simulink model "hydraulic_actuator"  (R2019b)
settings: Solver=ode23t  StartTime=0.0  StopTime=10.0  MaxStep=0.001  RelTol=1e-6  EnableMultiTasking=on
libraries: simulink x1
Description:
  | Closed-Loop Electrohydraulic Actuator with Proportional Valve
  | 
  | This example shows an actuator that consists of a proportional 4-way directional valve
  | driving a double-acting hydraulic cylinder. The cylinder drives a load consisting of a mass,
  | viscous and Coulomb friction, constant force, and a spring. The actuator is powered
  | by a variable-displacement, pressure-compensated pump, driven by a constant velocity
  | motor. Pipelines between the valve, cylinder, pump, and the tank are simulated
  | with the Hydraulic Pipeline blocks.
  | 
  | 
  | Copyright 2008-2013 The MathWorks, Inc.
settings Model: DataDictionary=HeliSystemDD.sldd  ExtModeAutoUpdateStatusClock=off  Creator=MathWorks  LastModifiedBy=bpotter
settings DataIOCC: LimitDataPoints=on  SaveFormat=Array  SaveOutput=off  SignalLogging=off  DSMLogging=off  SaveTime=off  ReturnWorkspaceOutputs=off
settings OptimizationCC: DefaultParameterBehavior=Inlined  UseDivisionForNetSlopeComputation=on  ExpressionDepthLimit=2147483647  InitFltsAndDblsToZero=on  LifeSpan=inf
settings DebuggingCC: SaveWithParameterizedLinksMsg=none  SignalResolutionControl=TryResolveAllWithWarning  SolverPrmCheckMsg=warning  MultiTaskDSMMsg=warning  ParameterPrecisionLossMsg=none  AllowSymbolicDim=off  StateNameClashWarn=warning  PregeneratedLibrarySubsystemCodeDiagnostic=none  StrictBusMsg=ErrorOnBusTreatedAsVector  NonBusSignalsTreatedAsBus=error  SFUnexpectedBacktrackingDiag=warning  SFNoUnconditionalDefaultTransitionDiag=warning  SFExecutionAtInitializationDiag=none  ArithmeticOperatorsInVariantConditions=warning
settings HardwareCC: ProdBitPerPointer=32  ProdBitPerSizeT=32  ProdBitPerPtrDiffT=32  ProdLargestAtomicFloat=None  ProdEndianess=Unspecified  ProdWordSize=32  ProdHWDeviceType=32-bit Generic
settings ModelReferenceCC: PropagateSignalLabelsOutOfModel=off
settings SFSimCC: SimUseLocalCustomCode=off  CustomCodeUndefinedFunction=UseInterfaceOnly
settings RTWCC: RTWUseLocalCustomCode=off
settings CodeAppCC: StateflowObjectComments=on
settings GRTTargetCC: TargetFcnLib=ansi_tfl_tmw.mat  TargetLangStandard=C89/C90 (ANSI)  GeneratePreprocessorConditionals=Disable all  CombineOutputUpdateFcns=off  GRTInterface=on
settings ConfigComp: CovMetricSettings=dw  CovHtmlReporting=on  CovSaveCumulativeToWorkspaceVar=on  CovSaveSingleToWorkspaceVar=on  CovExternalEMLEnable=off  CovSFcnEnable=off
settings SimscapeCC: SimscapeNormalizeSystem=off

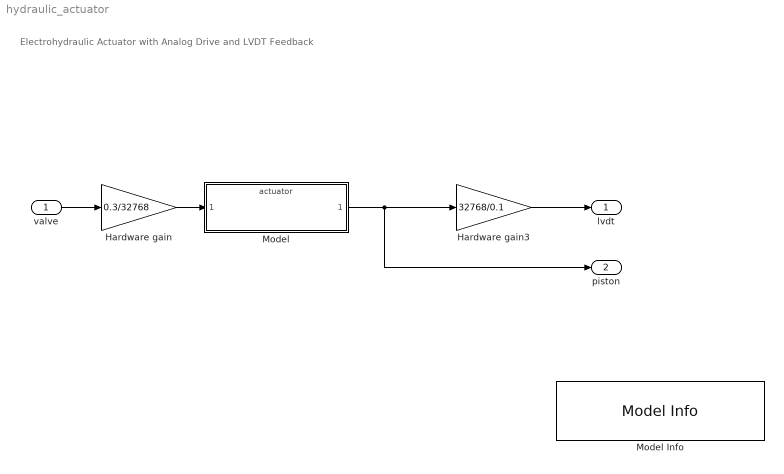
== system hydraulic_actuator ==
  note: Electrohydraulic Actuator with Analog Drive and LVDT Feedback
  valve : Inport  OutDataTypeStr=int16  PortDimensions=1  SampleTime=0.001
  Hardware gain : Gain  Gain=0.3/32768  OutDataTypeStr=double
  Hardware gain3 : Gain  Gain=32768/0.1  OutDataTypeStr=int16  SaturateOnIntegerOverflow=on
  Model : ModelReference  ModelNameDialog=actuator  SimulationMode=Normal  ModelReferenceVersion=1.107
  Model Info : simulink/Model-Wide Utilities/Model Info  Frame=on  DisplayStringWithTags=|  HorizontalTextAlignment=Center  LeftAlignmentValue=0.5
      | Model: %<ModelName>
      | Model Version: %<ModelVersion>
      | Last Modified: %<LastModificationDate>
      | 
      | Copyright 2019 The MathWorks, Inc.
  lvdt : Outport  OutDataTypeStr=int16  PortDimensions=1  VectorParamsAs1DForOutWhenUnconnected=off
  piston : Outport  Port=2  OutDataTypeStr=double  PortDimensions=1  VectorParamsAs1DForOutWhenUnconnected=off
  wires:
  valve/1 -> Hardware gain/1
  Hardware gain/1 -> Model/1
  Model/1 -> piston/1, Hardware gain3/1
  Hardware gain3/1 -> lvdt/1
